simulink model "Serial_Motor"  (R2025b)
settings: Solver=ode4  StartTime=0.0  StopTime=inf  FixedStep=0.01  RelTol=1e-3
undefined symbols (not defined in the file or in its folder): LF
libraries: instrumentseriallib x3, sldrtlib x1
settings Model: Creator=joshc  LastModifiedBy=joshc
settings HardwareCC: ProdBitPerLong=64.0  ProdHWDeviceType=Intel->x86-64 (Linux 64)
settings RTWCC: SystemTargetFile=sldrt.tlc  TemplateMakefile=sldrt.tmf  RTWCompilerOptimization=on  Description=Simulink Desktop Real-Time
settings CodeAppCC: MaxIdLength=95.0
settings SimulinkDesktopRealTimeCC: ExtModeTransport=0.0  ExtModeStaticAllocSize=1000000.0  TargetLibSuffix=_sldrt.a  TargetPreCompLibLocation=C:\Program Files\MATLAB\R2025b\toolbox\sldrt\lib\win64  MultiwordLength=2048.0  DynamicStringBufferSize=256.0  ParMdlRefBuildCompliant=on  PreserveMATLABNamespacesInGeneratedCode=on  SubcomponentCodeInterfacePackaging=Reusable function

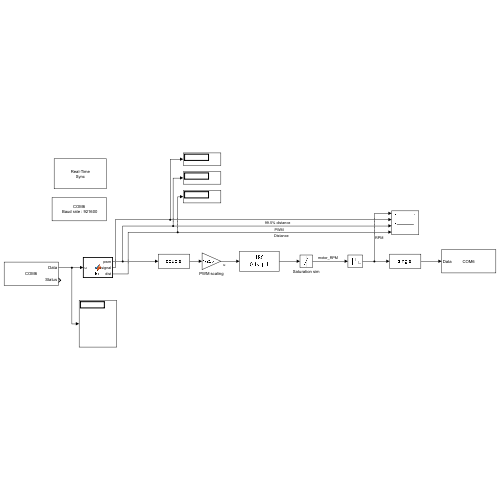
[thumbnail: Simulink's stored preview of the top-level diagram]
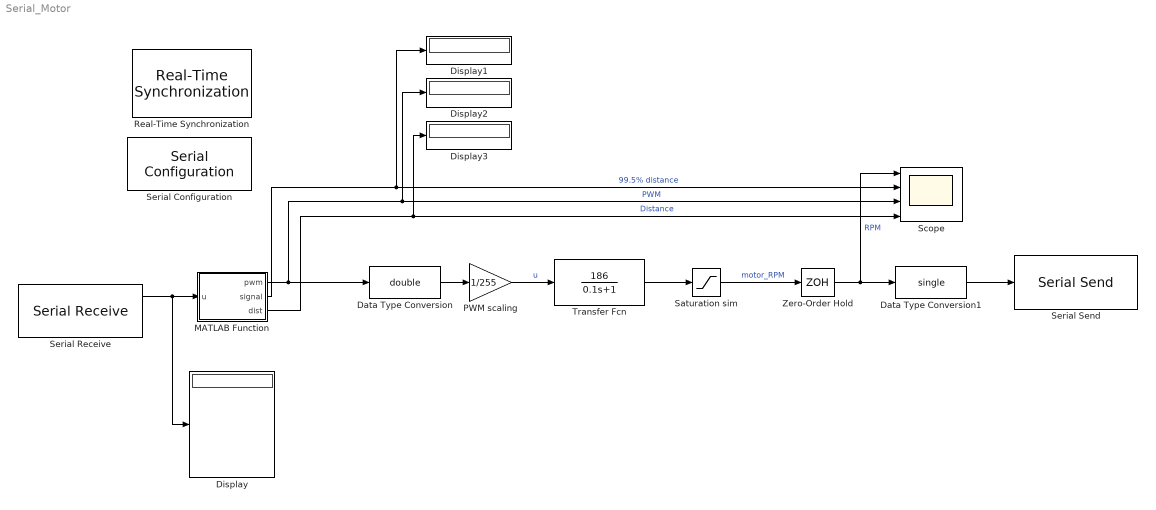
== system Serial_Motor ==
  Data Type Conversion : DataTypeConversion  OutDataTypeStr=double  SaturateOnIntegerOverflow=off  RndMeth=Floor
  Data Type Conversion1 : DataTypeConversion  OutDataTypeStr=single  SaturateOnIntegerOverflow=off  RndMeth=Floor
  Display{,1..3} (4 alike) : Display
  MATLAB Function : MATLAB Function  TreatAsAtomicUnit=on
  PWM scaling : Gain  Gain=1/255
  Real-Time Synchronization : sldrtlib/Real-Time Synchronization  SampleTime=0.01  MaxMissedTicks=2000  ShowMissedTicks=off  YieldWhenWaiting=on
  Saturation sim : Saturate  UpperLimit=186  LowerLimit=0
  Scope : Scope  NumInputPorts=4
      settings: TimeSpan=10  ActiveDisplayYMinimum=-1.451153051925585E+34  ActiveDisplayYMaximum=1.3060377467330254E+35
  Serial Configuration : instrumentseriallib/Serial Configuration  Priority=-200000  PortSel=COM6  Port=COM6  ComPort=COM6  BaudRate=921600  DataBits=8  Parity=none  StopBits=1  ByteOrder=little-endian  FlowControl=none  Timeout=10  SimulateUsing=Interpreted execution  BlockInModel=on  aMode=1
  Serial Receive : instrumentseriallib/Serial Receive  Priority=1  PortSel=COM6  Port=COM6  ComPort=COM6  DataType=uint8  SaveDataType=uint8  ToggleHeader=on  Header=[187]  ToggleDataSize=on  DataSize=[6, 1]  ToggleTerminator=off  Terminator=LF ('\n')  CustomTerminator=[]  InputFormat=Column major  EnableBlockingMode=off  ActionDataUnavailable=Output last received value  ActionWhenDataUnavailable=Output last received value  CustomValue=0  SampleTime=0.01  SimulateUsing=Interpreted execution  BlockInModel=on  aMode=1  LibraryInUse=instrumentlib
  Serial Send : instrumentseriallib/Serial Send  Priority=1  PortSel=COM6  Port=COM6  ComPort=COM6  Header=[]  Terminator=<none>  CustomTerminator=[]  EnableBlockingMode=off  SimulateUsing=Interpreted execution  BlockInModel=on  aMode=1
  Transfer Fcn : TransferFcn  Numerator=[186]  Denominator=[0.1 1]
  Zero-Order Hold : ZeroOrderHold  SampleTime=0.01
  wires:
  PWM scaling/1 -> Transfer Fcn/1  "u"
  Transfer Fcn/1 -> Saturation sim/1
  Saturation sim/1 -> Zero-Order Hold/1  "motor_RPM"
  Zero-Order Hold/1 -> Data Type Conversion1/1, Scope/1  "RPM"
  Data Type Conversion/1 -> PWM scaling/1
  Data Type Conversion1/1 -> Serial Send/1
  MATLAB Function/1(pwm) -> Data Type Conversion/1, Scope/3, Display2/1  "PWM"
  MATLAB Function/2(signal) -> Scope/2, Display1/1  "99.5% distance"
  Serial Receive/1 -> Display/1, MATLAB Function/1(u)
  MATLAB Function/3(dist) -> Scope/4, Display3/1  "Distance"

== matlab function Serial_Motor/MATLAB Function ==
  data: u input; pwm output; signal output; dist output
function [pwm, signal, dist] = fcn(u)
    % Initialize outputs to ensure they are scalars
    pwm    = 0;
    signal = 0;
    dist   = single(0);

    % Use coder.varsize to tell Simulink u might be variable (safety)
    % but we treat it as fixed length 6
    if length(u) == 6
        pwm    = double(u(1));
        signal = double(u(2));
        
        % Typecast the float bytes
        % We extract u(3:6) and force it to be a scalar single
        temp_dist = typecast(u(3:6), 'single');
        dist = temp_dist(1); 
    end
end
